simulink model "feedbackImpedanceJoints"  (R2018a)
settings: Solver=FixedStepAuto  StartTime=0.0  StopTime=100.0  RelTol=1e-3
libraries: dspnetwork x2, dspsrcs4 x2, sldrtlib x1
settings Model: Creator=ronnie  LastModifiedBy=user

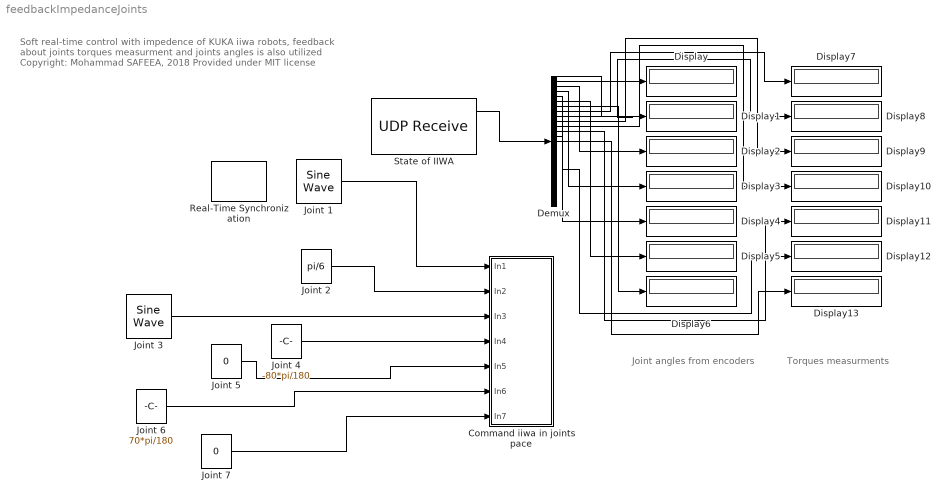
== system feedbackImpedanceJoints ==
  note: Torques measurments
  note: Joint angles from encoders
  note: Soft real-time control with impedence of KUKA iiwa robots,
      | feedback about joints torques measurment and joints angles
      | is also utilized
      |
      | Copyright: Mohammad SAFEEA, 2018
      | Provided under MIT license
  Command iiwa in joints pace : Subsystem
  Demux : Demux  Outputs=21+6
  Display{,1..13} (14 alike) : Display
  Joint 1 : dspsrcs4/Sine Wave  Amplitude=0.25  Frequency=0.15  Phase=0  SampleMode=Discrete  OutComplex=Real  CompMethod=Trigonometric fcn  TableSize=Speed  SampleTime=1/1000  SamplesPerFrame=1  ResetState=Restart at time zero  OutputFrames=off  dataType=double  wordLen=16  udDataType=sfix(16)  fracBitsMode=Best precision  numFracBits=15  OutDataTypeStr=double  LastOutDataTypeStr=double
  Joint 2 : Constant  Value=pi/6  VectorParams1D=off  SampleTime=1/1000
  Joint 3 : dspsrcs4/Sine Wave  Amplitude=0.35  Frequency=0.15  Phase=0  SampleMode=Discrete  OutComplex=Real  CompMethod=Trigonometric fcn  TableSize=Speed  SampleTime=1/1000  SamplesPerFrame=1  ResetState=Restart at time zero  OutputFrames=off  dataType=double  wordLen=16  udDataType=sfix(16)  fracBitsMode=Best precision  numFracBits=15  OutDataTypeStr=double  LastOutDataTypeStr=double
  Joint 4 : Constant  Value=-80*pi/180  VectorParams1D=off  SampleTime=1/1000
  Joint 5 : Constant  Value=0  VectorParams1D=off  SampleTime=1/1000
  Joint 6 : Constant  Value=70*pi/180  VectorParams1D=off  SampleTime=1/1000
  Joint 7 : Constant  Value=0  VectorParams1D=off  SampleTime=1/1000
  Real-Time Synchronization : sldrtlib/Real-Time Synchronization  SampleTime=0.01  MaxMissedTicks=10  ShowMissedTicks=off  YieldWhenWaiting=off
  State of IIWA : dspnetwork/UDP Receive  localURL='0.0.0.0'  localPort=30008  remoteURL='172.31.1.147'  remotePort=-1  recvBufferSize=8192  dims=21+6  signalDatatype=double  isVarSize=off  showBlockingTime=off  blockingTime=0  sampletime=0.01  blockPlatform=[]
      settings: SourceProductName=DSP System Toolbox  SourceProductBaseCode=DS
  wires:
  Joint 1/1 -> Command iiwa in joints pace/1(In1)
  Joint 2/1 -> Command iiwa in joints pace/2(In2)
  Joint 3/1 -> Command iiwa in joints pace/3(In3)
  Joint 4/1 -> Command iiwa in joints pace/4(In4)
  Joint 5/1 -> Command iiwa in joints pace/5(In5)
  Joint 7/1 -> Command iiwa in joints pace/7(In7)
  Joint 6/1 -> Command iiwa in joints pace/6(In6)
  Demux/1 -> Display/1
  Demux/7 -> Display6/1
  Demux/13 -> Display12/1
  Demux/3 -> Display2/1
  Demux/9 -> Display8/1
  Demux/11 -> Display10/1
  Demux/10 -> Display9/1
  Demux/6 -> Display5/1
  Demux/4 -> Display3/1
  Demux/8 -> Display7/1
  Demux/12 -> Display11/1
  Demux/14 -> Display13/1
  Demux/2 -> Display1/1
  State of IIWA/1 -> Demux/1
  Demux/5 -> Display4/1

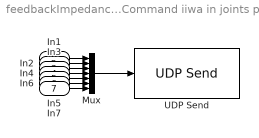
== system feedbackImpedanceJoints/Command iiwa in joints pace ==
  In1 : Inport
  In2 : Inport  Port=2
  In3 : Inport  Port=3
  In4 : Inport  Port=4
  In5 : Inport  Port=5
  In6 : Inport  Port=6
  In7 : Inport  Port=7
  Mux : Mux  Inputs=7
  UDP Send : dspnetwork/UDP Send  remoteURL='172.31.1.147'  remotePort=30002  localURL='0.0.0.0'  localPortSource=Automatically determine  localPort=-1  sampletime=-1  blockPlatform=[]  separateLengthPort=0
      settings: SourceProductName=DSP System Toolbox  SourceProductBaseCode=DS
  wires:
  Mux/1 -> UDP Send/1
  In3/1 -> Mux/3
  In5/1 -> Mux/5
  In2/1 -> Mux/2
  In1/1 -> Mux/1
  In6/1 -> Mux/6
  In4/1 -> Mux/4
  In7/1 -> Mux/7
